simulink model "SetResetOut"  (Simulink 5.0)
settings: Solver=FixedStepDiscrete  StartTime=0.0  StopTime=10000.0  RelTol=1e-3
libraries: simulink x2
settings Model: Creator=scaife  LastModifiedBy=scaife  ExtModeAutoUpdateStatusClock=off

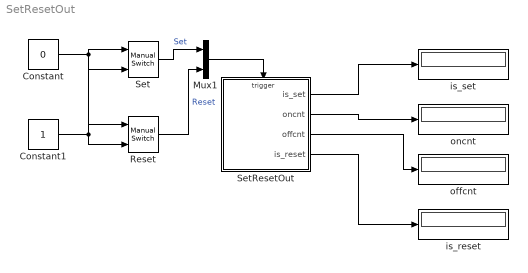
== system SetResetOut ==
  Constant : Constant  Value=0
  Constant1 : Constant
  Mux1 : Mux  Inputs=2
  Reset : simulink/Signal Routing/Manual Switch  sw=1  action=0
  Set : simulink/Signal Routing/Manual Switch  sw=1  action=0
  SetResetOut : Stateflow chart
  is_reset : Display
  is_set : Display
  offcnt : Display
  oncnt : Display
  wires:
  Mux1/1 -> SetResetOut/Trigger
  Constant/1 -> Set/1, Reset/1
  Constant1/1 -> Reset/2, Set/2
  Set/1 -> Mux1/1  "Set"
  Reset/1 -> Mux1/2  "Reset"
  SetResetOut/4(is_reset) -> is_reset/1
  SetResetOut/3(offcnt) -> offcnt/1
  SetResetOut/2(oncnt) -> oncnt/1
  SetResetOut/1(is_set) -> is_set/1

== stateflow chart SetResetOut ==
  state On/
    en: is_set=1; oncnt++;
    du: oncnt++;
    ex: is_reset=1;
  state Off/
    en: is_set=2; offcnt++;
    du: offcnt++;
    ex: is_reset=2;
  (default) -> Off
  On -> Off : Reset
  Off -> On : Set
  data: is_set output int32; oncnt output int32; offcnt output int32; is_reset output int32
  events: Set input EITHER_EDGE_EVENT; Reset input EITHER_EDGE_EVENT
